simulink model "ex6_2a2"  (Simulink 7.5)
settings: Solver=ode45  StartTime=0.0  StopTime=0.04  RelTol=1e-3
values from neighbouring files (symbols this model uses):
  alpha = 0:0.01:180    [ex6_2b.m]
undefined symbols (not defined in the file or in its folder): E, L, R
libraries: powerlib x15
settings Model: Creator=107108103  LastModifiedBy=Sambhav
settings OptimizationCC: InitFltsAndDblsToZero=on
settings DebuggingCC: StrictBusMsg=Warning

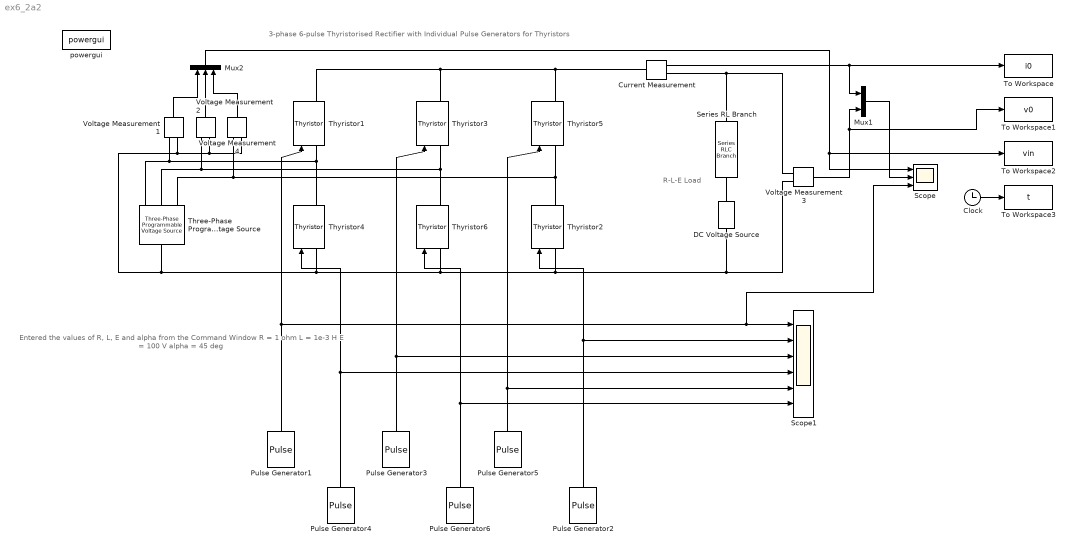
== system ex6_2a2 ==
  note: R-L-E Load
  note: 3-phase 6-pulse Thyristorised Rectifier with Individual Pulse Generators for Thyristors
  note: Entered the values of
      | R, L, E and alpha from
      | the Command Window
      | R = 1 ohm
      | L = 1e-3 H
      | E = 100 V
      | alpha = 45 deg
  Clock : Clock
      settings: Decimation=10
  Current Measurement : powerlib/Measurements/Current Measurement  DialogController=POWERSYS.PowerSysDialog  SystemSampleTime=-1  PhasorSimulation=off  OutputType=Complex  PSBequivalent=0
  DC Voltage Source : powerlib/Electrical Sources/DC Voltage Source  DialogController=POWERSYS.PowerSysDialog  SystemSampleTime=-1  Amplitude=E  Measurements=None
  Mux1 : Mux  Inputs=2
  Mux2 : Mux  Inputs=3
  Pulse Generator1 : DiscretePulseGenerator  PulseType=Time based  Amplitude=1  Period=20e-3  PulseWidth=2  PhaseDelay=((alpha+30)*10/180)*1e-3  SampleTime=1
  Pulse Generator2 : DiscretePulseGenerator  PulseType=Time based  Amplitude=1  Period=20e-3  PulseWidth=2  PhaseDelay=((alpha+90)*10/180)*1e-3  SampleTime=1
  Pulse Generator3 : DiscretePulseGenerator  PulseType=Time based  Amplitude=1  Period=20e-3  PulseWidth=2  PhaseDelay=((alpha+150)*10/180)*1e-3  SampleTime=1
  Pulse Generator4 : DiscretePulseGenerator  PulseType=Time based  Amplitude=1  Period=20e-3  PulseWidth=2  PhaseDelay=((alpha+210)*10/180)*1e-3  SampleTime=1
  Pulse Generator5 : DiscretePulseGenerator  PulseType=Time based  Amplitude=1  Period=20e-3  PulseWidth=2  PhaseDelay=((alpha+270)*10/180)*1e-3  SampleTime=1
  Pulse Generator6 : DiscretePulseGenerator  PulseType=Time based  Amplitude=1  Period=20e-3  PulseWidth=2  PhaseDelay=((alpha+330)*10/180)*1e-3  SampleTime=1
  Scope : Scope  NumInputPorts=3
      settings: YMin=-5~-5~-5  YMax=5~5~5
  Scope1 : Scope  NumInputPorts=6
      settings: YMin=-5~-5~-5~-5~-5~-5  YMax=5~5~5~5~5~5
  Series RL Branch : powerlib/Elements/Series RLC Branch  DialogController=POWERSYS.PowerSysDialog  PhysicalDomain=powersysdomain  SubClassName=unknown  LeftPortType=p1  RightPortType=p1  LConnTagsString=__new0  RConnTagsString=__new0  BranchType=RL  Resistance=R  Inductance=L  SetiL0=off  InitialCurrent=0  Capacitance=1.0  Setx0=off  InitialVoltage=0  Measurements=None
  Three-Phase Programmable Voltage Source : powerlib/Electrical Sources/Three-Phase Programmable Voltage Source  DialogController=POWERSYS.PowerSysDialog  SystemSampleTime=-1  PositiveSequence="[415  0 50]"  VariationEntity=None  VariationType=Step  VariationStep=0.5  VariationRate=10  VariationMagnitude=0.3  VariationFrequency=2  VariationTiming=[1 2]  VariationPhaseA=off  Amplitudes=[1 0.8 1.2 1.0]  TimeValues=[0 0.1 0.15 0.2]  HarmonicGeneration=off  HarmonicA=[3 0.2 -25 0]  HarmonicB=[2 0.15 35 2]  Timing="[0.05  3]"
  Thyristor{1..6} (6 alike) : powerlib/Power Electronics/Thyristor  DialogController=POWERSYS.PowerSysDialog  SystemSampleTime=-1  Ron=0.001  Lon=0  Vf=0.8  IC=0  Rs=500  Cs=250e-9  Measurements=on
  To Workspace : ToWorkspace  VariableName=i0  SampleTime=-1  SaveFormat=Array
  To Workspace1 : ToWorkspace  VariableName=v0  SampleTime=-1  SaveFormat=Array
  To Workspace2 : ToWorkspace  VariableName=vin  SampleTime=-1  SaveFormat=Array
  To Workspace3 : ToWorkspace  VariableName=t  SampleTime=-1  SaveFormat=Array
  Voltage Measurement{1..4} (4 alike) : powerlib/Measurements/Voltage Measurement  DialogController=POWERSYS.PowerSysDialog  SystemSampleTime=-1  PhasorSimulation=off  OutputType=Complex  PSBequivalent=0
  powergui : powerlib/powergui  SystemSampleTime=-1  SimulationMode=Continuous  SampleTime=50e-6  frequency=60  SPID=off  DisableSnubberDevices=off  DisableRonSwitches=off  DisableVfSwitches=off  SwTol=0  Interpol=off  frequencyindice=50  echomessages=off  HookPort=off  DisplayEquations=off  FunctionMessages=off  EnableUseOfTLC=off  x0status=blocks  RestoreLinks=warning  ResistiveCurrentMeasurement=off  Frange=[0:2:500]  Ylog=off  Xlog=on  ShowGrid=off  save=off  variable=ZData  ZoomFFT=on  StartTime=0.0  cycles=1  DisplayStyle=1  fundamental=60  FreqAxis=off  MaxFrequency=1000  frequencyindicesteady=1  RmsSteady=1  display=off  Ts=0  methode=off
  wires:
  Pulse Generator1/1 -> Thyristor1/1, Scope1/1, Scope/3
  Pulse Generator2/1 -> Thyristor2/1, Scope1/2
  Pulse Generator3/1 -> Thyristor3/1, Scope1/3
  Pulse Generator4/1 -> Thyristor4/1, Scope1/4
  Pulse Generator6/1 -> Thyristor6/1, Scope1/6
  Pulse Generator5/1 -> Thyristor5/1, Scope1/5
  Voltage Measurement1/1 -> Mux2/1
  Voltage Measurement2/1 -> Mux2/2
  Voltage Measurement4/1 -> Mux2/3
  Mux2/1 -> Scope/1, To Workspace2/1
  Current Measurement/1 -> Mux1/1, To Workspace/1
  Voltage Measurement3/1 -> Mux1/2, To Workspace1/1
  Mux1/1 -> Scope/2
  Clock/1 -> To Workspace3/1
  connections:
  Three-Phase Programmable Voltage Source/RConn1 -- Voltage Measurement1/LConn1 -- Thyristor4/RConn1 -- Thyristor1/LConn1
  Three-Phase Programmable Voltage Source/RConn2 -- Thyristor3/LConn1 -- Thyristor6/RConn1 -- Voltage Measurement2/LConn1
  Three-Phase Programmable Voltage Source/RConn3 -- Thyristor2/RConn1 -- Thyristor5/LConn1 -- Voltage Measurement4/LConn1
  Voltage Measurement3/LConn1 -- Series RL Branch/LConn1 -- Current Measurement/RConn1
  DC Voltage Source/RConn1 -- Series RL Branch/RConn1
  Thyristor5/RConn1 -- Thyristor1/RConn1 -- Thyristor3/RConn1 -- Current Measurement/LConn1
  Voltage Measurement1/LConn2 -- Voltage Measurement4/LConn2 -- Voltage Measurement2/LConn2 -- Thyristor2/LConn1 -- DC Voltage Source/LConn1 -- Voltage Measurement3/LConn2 -- Thyristor6/LConn1 -- Thyristor4/LConn1 -- Three-Phase Programmable Voltage Source/LConn1
